simulink model "blowerControlBall"  (R2022b)
settings: Solver=ode1  StartTime=0.0  StopTime=100  FixedStep=0.001  RelTol=1e-3
values from neighbouring files (symbols this model uses):
  A = 1/(4*tita*tita*sqrt(2))    [controllerId.m]    (also in identif_tf.m = 0.00679290871522)
  Cd = 1    [identif_tf.m]
  g = 9.8    [identif_tf.m]
  Hcs1 = minreal(Hds1/Hf1)    [controllerId.m]
  m = 2.7/1000    (= 0.0027)    [identif_tf.m]
  pwm_values = [0 20 60 100]    [identif_tf.m]
  q_points = [0 0.5 1.3 1.55]    [identif_tf.m]
  ro = 1.225    [identif_tf.m]
  Vb = (4*pi*(d_ball/2)^3)/3    (= 2.24492975038e-05)    [identif_tf.m]
settings Model: Creator=Admin  LastModifiedBy=Admin

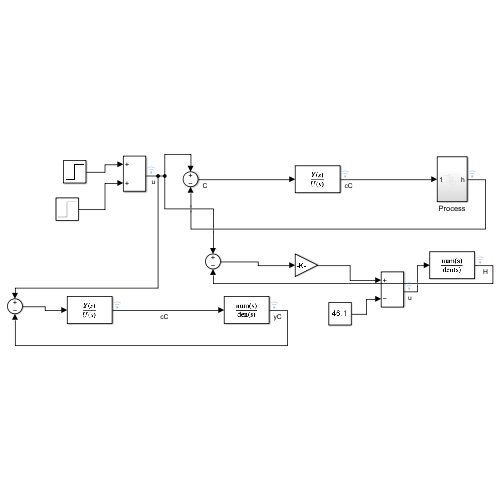
[thumbnail: Simulink's stored preview of the top-level diagram]
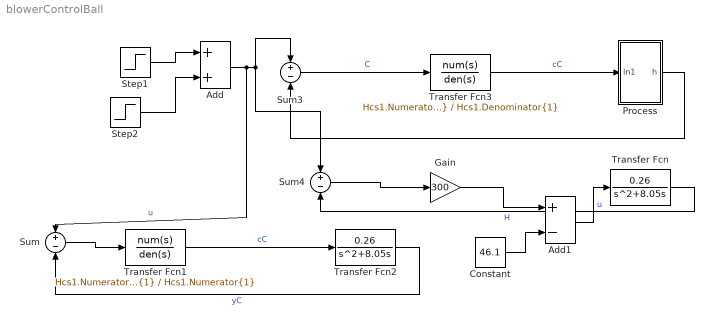
== system blowerControlBall ==
  Add : Sum
  Add1 : Sum  Inputs=+-
  Constant : Constant  Value=46.1
  Gain : Gain  Gain=300
  Process : Subsystem
  Step1 : Step  Time=0  After=0.3  SampleTime=0
  Step2 : Step  Time=10  After=0.1  SampleTime=0
  Sum : Sum  Inputs=+-
  Sum3 : Sum  Inputs=+-
  Sum4 : Sum  Inputs=+-
  Transfer Fcn : TransferFcn  Numerator=[0.26]  Denominator=[1 8.05 0]
  Transfer Fcn1 : TransferFcn  Numerator=Hcs1.Numerator{1}  Denominator=Hcs1.Numerator{1}
  Transfer Fcn2 : TransferFcn  Numerator=[0.26]  Denominator=[1 8.05 0]
  Transfer Fcn3 : TransferFcn  Numerator=Hcs1.Numerator{1}  Denominator=Hcs1.Denominator{1}
  wires:
  Step1/1 -> Add/1
  Add/1 -> Sum/1, Sum4/1, Sum3/1  "u"
  Step2/1 -> Add/2
  Process/1(h) -> Sum3/2
  Transfer Fcn/1 -> Sum4/2  "H"
  Sum4/1 -> Gain/1
  Gain/1 -> Add1/1
  Transfer Fcn1/1 -> Transfer Fcn2/1  "cC"
  Sum/1 -> Transfer Fcn1/1
  Transfer Fcn2/1 -> Sum/2  "yC"
  Add1/1 -> Transfer Fcn/1  "u"
  Constant/1 -> Add1/2
  Sum3/1 -> Transfer Fcn3/1  "C"
  Transfer Fcn3/1 -> Process/1(In1)  "cC"

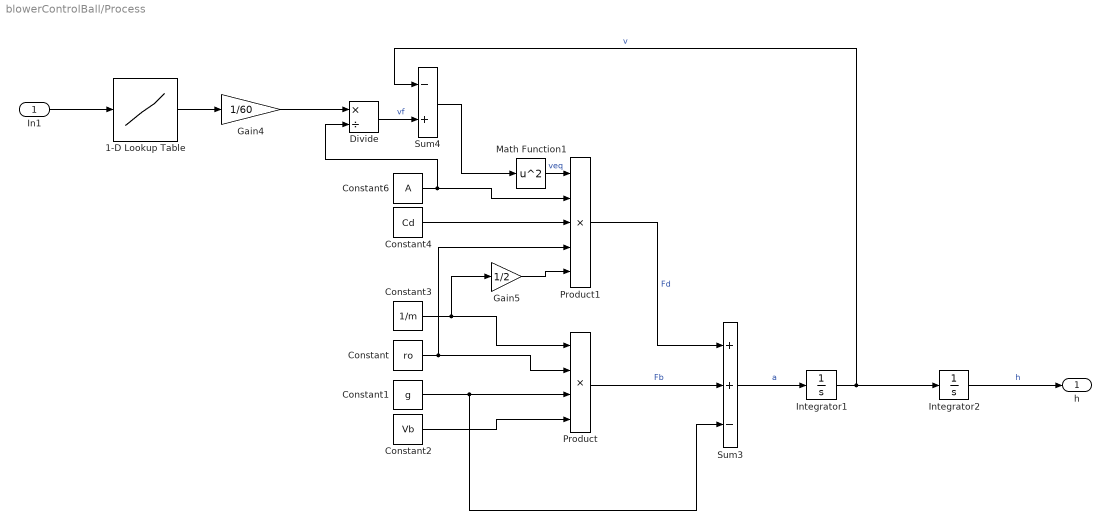
== system blowerControlBall/Process ==
  In1 : Inport
  1-D Lookup Table : Lookup_n-D  NumberOfTableDimensions=1  BreakpointsForDimension1=pwm_values  Table=q_points  InternalRulePriority=Speed  RndMeth=Simplest
  Constant : Constant  Value=ro
  Constant1 : Constant  Value=g
  Constant2 : Constant  Value=Vb
  Constant3 : Constant  Value=1/m
  Constant4 : Constant  Value=Cd
  Constant6 : Constant  Value=A
  Divide : Product  Inputs=*/
  Gain4 : Gain  Gain=1/60
  Gain5 : Gain  Gain=1/2
  Integrator1 : Integrator
  Integrator2 : Integrator
  Math Function1 : Math  Operator=square
  Product : Product  Inputs=4
  Product1 : Product  Inputs=5
  Sum3 : Sum  Inputs=++-
  Sum4 : Sum  Inputs=-+
  h : Outport
  wires:
  Constant/1 -> Product1/4, Product/2
  Constant6/1 -> Divide/2, Product1/2
  Integrator1/1 -> Sum4/1, Integrator2/1  "v"
  Math Function1/1 -> Product1/1  "veq"
  Constant3/1 -> Gain5/1, Product/1
  Product/1 -> Sum3/2  "Fb"
  Constant4/1 -> Product1/3
  Integrator2/1 -> h/1  "h"
  Gain5/1 -> Product1/5
  Sum3/1 -> Integrator1/1  "a"
  Sum4/1 -> Math Function1/1
  Gain4/1 -> Divide/1
  Constant1/1 -> Sum3/3, Product/3
  Constant2/1 -> Product/4
  Product1/1 -> Sum3/1  "Fd"
  Divide/1 -> Sum4/2  "vf"
  1-D Lookup Table/1 -> Gain4/1
  In1/1 -> 1-D Lookup Table/1
